simulink model "APB_Model0_v03_Test"  (R2020b)
settings: Solver=ode45  StartTime=0.0  StopTime=inf  RelTol=1e-3
undefined symbols (not defined in the file or in its folder): calb_Driver_acce, calb_Driver_bttn, calb_Driver_EmrBrk, calb_Driver_Prss, G_Fclamp, G_Kmot, G_Rmot, G_Stroke, G_SwOmega, GEN3, PbcDataStorageRequest_t
libraries: etargetslib x26, Lib_Op_Hndl x4, simulink x2, PbcOut_Checksum x2
(part 4 of 5)

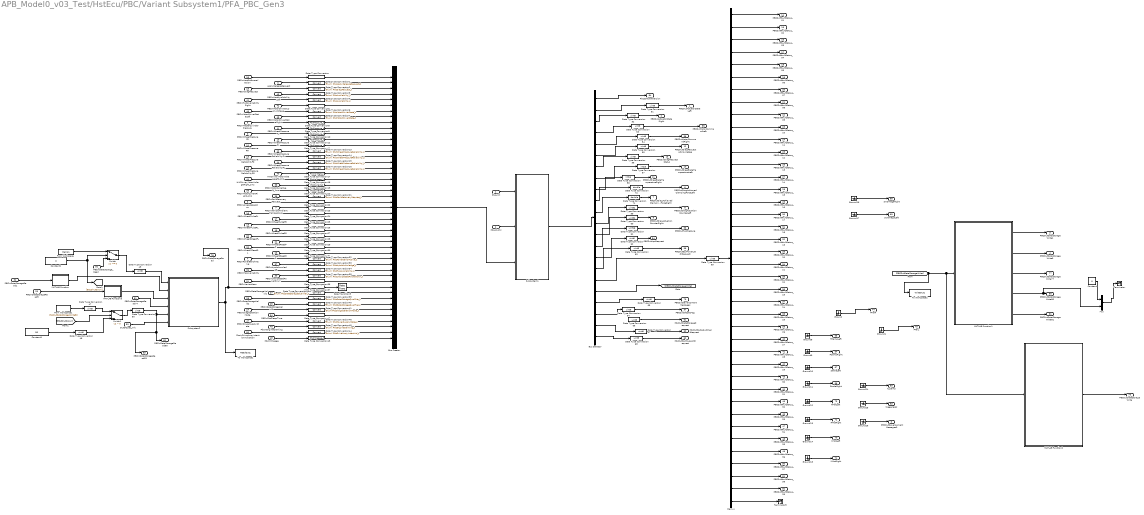
== system APB_Model0_v03_Test/HstEcu/PBC/Variant Subsystem1/PFA_PBC_Gen3 ==
  Pbc_Init : Inport
  Pbc_Cyclic : Inport  Port=2
  ApplyReleaseRequest : Inport  Port=3
      settings: AttributesFormatString=|
      | Type : %<OutDataTypeStr>
      | Unit : %<Unit>
  PBCInRollerBenchActive : Inport  Port=4
      settings: AttributesFormatString=|
      | Type : %<OutDataTypeStr>
      | Unit : %<Unit>
  PBCInLongAcceleration : Inport  Port=5
      settings: AttributesFormatString=|
      | Type : %<OutDataTypeStr>
      | Unit : %<Unit>
  PBCInMasterCylinderPressure : Inport  Port=6
      settings: AttributesFormatString=|
      | Type : %<OutDataTypeStr>
      | Unit : %<Unit>
  PBCInVehicleAmbientTemperature : Inport  Port=7
      settings: AttributesFormatString=|
      | Type : %<OutDataTypeStr>
      | Unit : %<Unit>
  PBCInWheelPressureFL : Inport  Port=8
      settings: AttributesFormatString=|
      | Type : %<OutDataTypeStr>
      | Unit : %<Unit>
  PBCInWheelPressureFR : Inport  Port=9
      settings: AttributesFormatString=|
      | Type : %<OutDataTypeStr>
      | Unit : %<Unit>
  PBCInWheelPressureRL : Inport  Port=10
      settings: AttributesFormatString=|
      | Type : %<OutDataTypeStr>
      | Unit : %<Unit>
  PBCInWheelPressureRR : Inport  Port=11
      settings: AttributesFormatString=|
      | Type : %<OutDataTypeStr>
      | Unit : %<Unit>
  PBCInWheelPressureReliabilityFL : Inport  Port=12
      settings: AttributesFormatString=|
      | Type : %<OutDataTypeStr>
      | Unit : %<Unit>
  PBCInWheelPressureReliabilityFR : Inport  Port=13
      settings: AttributesFormatString=|
      | Type : %<OutDataTypeStr>
      | Unit : %<Unit>
  PBCInWheelPressureReliabilityRL : Inport  Port=14
      settings: AttributesFormatString=|
      | Type : %<OutDataTypeStr>
      | Unit : %<Unit>
  PBCInWheelPressureReliabilityRR : Inport  Port=15
      settings: AttributesFormatString=|
      | Type : %<OutDataTypeStr>
      | Unit : %<Unit>
  PBCInWheelPulseFL : Inport  Port=16
      settings: AttributesFormatString=|
      | Type : %<OutDataTypeStr>
      | Unit : %<Unit>
  PBCInWheelPulseFR : Inport  Port=17
      settings: AttributesFormatString=|
      | Type : %<OutDataTypeStr>
      | Unit : %<Unit>
  PBCInWheelPulseRL : Inport  Port=18
      settings: AttributesFormatString=|
      | Type : %<OutDataTypeStr>
      | Unit : %<Unit>
  PBCInWheelPulseRR : Inport  Port=19
      settings: AttributesFormatString=|
      | Type : %<OutDataTypeStr>
      | Unit : %<Unit>
  PBCInWheelSPeedFL : Inport  Port=20
      settings: AttributesFormatString=|
      | Type : %<OutDataTypeStr>
      | Unit : %<Unit>
  PBCInWheelSPeedFR : Inport  Port=21
      settings: AttributesFormatString=|
      | Type : %<OutDataTypeStr>
      | Unit : %<Unit>
  PBCInWheelSPeedRL : Inport  Port=22
      settings: AttributesFormatString=|
      | Type : %<OutDataTypeStr>
      | Unit : %<Unit>
  PBCInWheelSPeedRR : Inport  Port=23
      settings: AttributesFormatString=|
      | Type : %<OutDataTypeStr>
      | Unit : %<Unit>
  PBCInDiagOperationMode : Inport  Port=24
      settings: AttributesFormatString=|
      | Type : %<OutDataTypeStr>
      | Unit : %<Unit>
  PBCInDiagRequest : Inport  Port=25
      settings: AttributesFormatString=|
      | Type : %<OutDataTypeStr>
      | Unit : %<Unit>
  PBCinHostSoftwareVersion : Inport  Port=26
      settings: AttributesFormatString=|
      | Type : %<OutDataTypeStr>
      | Unit : %<Unit>
  PBCInDataStorageValid1 : Inport  Port=27
      settings: AttributesFormatString=|
      | Type : %<OutDataTypeStr>
      | Unit : %<Unit>
  PBCInDataStorageValid2 : Inport  Port=28
      settings: AttributesFormatString=|
      | Type : %<OutDataTypeStr>
      | Unit : %<Unit>
  PBCInDataStorageValid3 : Inport  Port=29
      settings: AttributesFormatString=|
      | Type : %<OutDataTypeStr>
      | Unit : %<Unit>
  PBCInUnexpectedPowerDown : Inport  Port=30
      settings: AttributesFormatString=|
      | Type : %<OutDataTypeStr>
      | Unit : %<Unit>
  PBCInVariantItem : Inport  Port=31
      settings: AttributesFormatString=|
      | Type : %<OutDataTypeStr>
      | Unit : %<Unit>
  PBCInDataStorageRead1 : Inport  Port=32
      settings: AttributesFormatString=|
      | Type : %<OutDataTypeStr>
      | Unit : %<Unit>
  PBCInDataStorageRead9 : Inport  Port=33
      settings: AttributesFormatString=|
      | Type : %<OutDataTypeStr>
      | Unit : %<Unit>
  PBCInPbcSleepTime : Inport  Port=34
      settings: AttributesFormatString=|
      | Type : %<OutDataTypeStr>
      | Unit : %<Unit>
  PBCInFaultRecoveryRequest : Inport  Port=35
      settings: AttributesFormatString=|
      | Type : %<OutDataTypeStr>
      | Unit : %<Unit>
  PBCInHpsAvailability : Inport  Port=36
      settings: AttributesFormatString=|
      | Type : %<OutDataTypeStr>
      | Unit : %<Unit>
  PBCInHpsAcknowledge : Inport  Port=37
      settings: AttributesFormatString=|
      | Type : %<OutDataTypeStr>
      | Unit : %<Unit>
  PBCInMotorCurrentLeft_1ms : Inport  Port=38
      settings: AttributesFormatString=|
      | Type : %<OutDataTypeStr>
      | Unit : %<Unit>
  PBCInMotorCurrentRight_1ms : Inport  Port=39
      settings: AttributesFormatString=|
      | Type : %<OutDataTypeStr>
      | Unit : %<Unit>
  HWDriver_MotorVoltageLeft_1ms : Inport  Port=40
      settings: AttributesFormatString=|
      | Type : %<OutDataTypeStr>
      | Unit : %<Unit>
  HWDriver_MotorVoltageRight_1ms : Inport  Port=41
      settings: AttributesFormatString=|
      | Type : %<OutDataTypeStr>
      | Unit : %<Unit>
  PBCInMotorDriverSupplyVoltage : Inport  Port=42
      settings: AttributesFormatString=|
      | Type : %<OutDataTypeStr>
      | Unit : %<Unit>
  PBCinHostAvailabilityLeft : Inport  Port=43
      settings: AttributesFormatString=|
      | Type : %<OutDataTypeStr>
      | Unit : %<Unit>
  PBCinHostAvailabilityRight : Inport  Port=44
      settings: AttributesFormatString=|
      | Type : %<OutDataTypeStr>
      | Unit : %<Unit>
  PBCInMotorDriverStateLeft : Inport  Port=45
      settings: AttributesFormatString=|
      | Type : %<OutDataTypeStr>
      | Unit : %<Unit>
  PBCInMotorDriverStateRight : Inport  Port=46
      settings: AttributesFormatString=|
      | Type : %<OutDataTypeStr>
      | Unit : %<Unit>
  PBCInPowerSupplyState : Inport  Port=47
      settings: AttributesFormatString=|
      | Type : %<OutDataTypeStr>
      | Unit : %<Unit>
  PbcInMileage : Inport  Port=48
      settings: AttributesFormatString=|
      | Type : %<OutDataTypeStr>
      | Unit : %<Unit>
  PbcInEngineCranking : Inport  Port=49
      settings: AttributesFormatString=|
      | Type : %<OutDataTypeStr>
      | Unit : %<Unit>
  PbcInDriveAwayIntentionIndication : Inport  Port=50
      settings: AttributesFormatString=|
      | Type : %<OutDataTypeStr>
      | Unit : %<Unit>
  PBCInDataStorageRead77 : Inport  Port=51
      settings: AttributesFormatString=|
      | Type : %<OutDataTypeStr>
      | Unit : %<Unit>
  PBCInDataStorage_Read : Inport  Port=52
      settings: AttributesFormatString=|
      | Type : %<OutDataTypeStr>
      | Unit : %<Unit>
  OutOfSpec_Init : Inport  Port=53
  Bus Creator : BusCreator  Inputs=47  OutDataTypeStr=Bus: PbcIn_t  NonVirtualBus=on
  Bus Selector : BusSelector  OutputSignals=PbcSoftwareVersion,ActuatorStateLeft,ActuatorStateRight,MotorCommandLeft,MotorCommandRight,DiagRequestAcknowledge,DiagRequestStatus,DiagBrakeTemperatureLeft,DiagBrakeTemperatureRight,DiagAchievedClampForceLeft,DiagAchievedClampForceRight,DiagActuationCounterLeft,DiagActuationCounterRight,HpsPressure,HpsRequest,EcuPowerLatchRequest,FaultStatus,DataStorageWrite,DevelopmentMessages,OutOfSpecMsg,PadAdjustmentRequest,ParkSupportRequest
  Constant : Constant  Value=0
  Constant1 : Constant  Value=50
  Constant2 : Constant  Value=0
  Data Type Conversion : DataTypeConversion  OutDataTypeStr=PbcVersionChar_t
  Data Type Conversion1 : DataTypeConversion  OutDataTypeStr=Enum: PbcApplyReleaseRequest_t
  Data Type Conversion{8..12} (5 alike) : DataTypeConversion  OutDataTypeStr=PbcPressure_t
  Data Type Conversion{13..16} (4 alike) : DataTypeConversion  OutDataTypeStr=Enum: PbcWheelPressureReliability_t
  Data Type Conversion17 : DataTypeConversion  OutDataTypeStr=PbcVoltage_t
  Data Type Conversion18 : DataTypeConversion  OutDataTypeStr=PbcVoltage_t
  Data Type Conversion19 : DataTypeConversion  OutDataTypeStr=PbcCurrent_t
  Data Type Conversion2 : DataTypeConversion  OutDataTypeStr=Enum: PbcDiagRequest_t
  Data Type Conversion20 : DataTypeConversion  OutDataTypeStr=PbcCurrent_t
  Data Type Conversion21 : DataTypeConversion  OutDataTypeStr=Enum: PbcFaultRecoveryRequest_t
  Data Type Conversion22 : DataTypeConversion  OutDataTypeStr=PbcAcceleration_t
  Data Type Conversion23 : DataTypeConversion  OutDataTypeStr=PbcTemperature_t
  Data Type Conversion{24..27} (4 alike) : DataTypeConversion  OutDataTypeStr=PbcWheelPulse_t
  Data Type Conversion{28..31} (4 alike) : DataTypeConversion  OutDataTypeStr=PbcWheelSpeed_t
  Data Type Conversion3 : DataTypeConversion  OutDataTypeStr=Enum: PbcAvailability_t
  Data Type Conversion32 : DataTypeConversion  OutDataTypeStr=Enum: PbcRollerbenchActive_t
  Data Type Conversion33 : DataTypeConversion  OutDataTypeStr=Enum: PbcHpsAcknowledge_t
  Data Type Conversion34 : DataTypeConversion  OutDataTypeStr=Enum: PbcHpsAvailability_t
  Data Type Conversion35 : DataTypeConversion  OutDataTypeStr=Enum: PbcUnexpectedPowerdown_t
  Data Type Conversion36 : DataTypeConversion  OutDataTypeStr=PbcVariantItem_t
  Data Type Conversion37 : DataTypeConversion  OutDataTypeStr=PbcDataStorage_t
  Data Type Conversion38 : DataTypeConversion  OutDataTypeStr=Enum: PbcDataStorageQualifier_t
  Data Type Conversion39 : DataTypeConversion  OutDataTypeStr=Enum: PbcDataStorageQualifier_t
  Data Type Conversion4 : DataTypeConversion  OutDataTypeStr=Enum: PbcAvailability_t
  Data Type Conversion40 : DataTypeConversion  OutDataTypeStr=Enum: PbcDataStorageQualifier_t
  Data Type Conversion41 : DataTypeConversion  OutDataTypeStr=Enum:PbcDiagOperationMode_t
  Data Type Conversion42 : DataTypeConversion  OutDataTypeStr=PbcSleepTime_t
  Data Type Conversion43 : DataTypeConversion  OutDataTypeStr=PbcMileage_t
  Data Type Conversion44 : DataTypeConversion  OutDataTypeStr=Enum: PbcDriveAwayIntentInd_t
  Data Type Conversion45 : DataTypeConversion  OutDataTypeStr=Enum: PbcEngineCranking_t
  Data Type Conversion46 : DataTypeConversion  OutDataTypeStr=Enum: PbcPowerSupplyState_t
  Data Type Conversion{47..56,62..69} (18 alike) : DataTypeConversion  OutDataTypeStr=uint8
  Data Type Conversion5 : DataTypeConversion  OutDataTypeStr=PbcDriverVoltage_t
  Data Type Conversion57 : DataTypeConversion  OutDataTypeStr=int16
  Data Type Conversion58 : DataTypeConversion  OutDataTypeStr=int16
  Data Type Conversion59 : DataTypeConversion  OutDataTypeStr=uint32
  Data Type Conversion6 : DataTypeConversion  OutDataTypeStr=Enum: PbcMotorDriverState_t
  Data Type Conversion60 : DataTypeConversion  OutDataTypeStr=uint32
  Data Type Conversion61 : DataTypeConversion  OutDataTypeStr=uint16
  Data Type Conversion7 : DataTypeConversion  OutDataTypeStr=Enum: PbcMotorDriverState_t
  Data Type Conversion70 : DataTypeConversion  OutDataTypeStr=double
  Data Type Conversion71 : DataTypeConversion  OutDataTypeStr=double
  Demux : Demux  Outputs=40
  From Workspace : FromWorkspace  VariableName=Memo1
  From Workspace1 : FromWorkspace  VariableName=PbcOutDataStorageWrite80
  Ground{,1,8..17,24..26} (15 alike) : Ground
  MATLAB Function : MATLAB Function  TreatAsAtomicUnit=on
  MATLAB Function1 : MATLAB Function  TreatAsAtomicUnit=on
  MATLAB Function2 : MATLAB Function  TreatAsAtomicUnit=on
  MATLAB Function3 : MATLAB Function  TreatAsAtomicUnit=on
  Mux : Mux  Inputs=2
  Rate Transition5 : RateTransition  OutPortSampleTime=0.01
      settings: AttributesFormatString=%<OutPortSampleTime>
  Subsystem1 : Subsystem
  Subsystem2 : Subsystem
  Switch : Switch  Criteria=u2 ~= 0
  Switch1 : Switch  Criteria=u2 > Threshold
  Terminator : Terminator
  Terminator3 : Terminator
  To Workspace1 : ToWorkspace  VariableName=ReadOut1  SaveFormat=Timeseries  SampleTime=-1
  To Workspace2 : ToWorkspace  VariableName=WriteOut1  SaveFormat=Timeseries  SampleTime=-1
  PBCOutActuatorStateLeft : Outport  VectorParamsAs1DForOutWhenUnconnected=off
      settings: AttributesFormatString=|
      | Type : %<OutDataTypeStr>\nInit :%<InitialOutput>
      | Unit : %<Unit>
  PBCOutActuatorStateRight : Outport  Port=2  VectorParamsAs1DForOutWhenUnconnected=off
      settings: AttributesFormatString=|
      | Type : %<OutDataTypeStr>\nInit :%<InitialOutput>
      | Unit : %<Unit>
  PBCOutDataStorageWrite1 : Outport  Port=3  VectorParamsAs1DForOutWhenUnconnected=off
      settings: AttributesFormatString=|
      | Type : %<OutDataTypeStr>\nInit :%<InitialOutput>
      | Unit : %<Unit>
  PBCOutDataStorageWrite9 : Outport  Port=4  VectorParamsAs1DForOutWhenUnconnected=off
      settings: AttributesFormatString=|
      | Type : %<OutDataTypeStr>\nInit :%<InitialOutput>
      | Unit : %<Unit>
  PBCOutDevelopmentMessages0 : Outport  Port=5  VectorParamsAs1DForOutWhenUnconnected=off
      settings: AttributesFormatString=|
      | Type : %<OutDataTypeStr>\nInit :%<InitialOutput>
      | Unit : %<Unit>
  PBCOutDiagAchievedClampingForceLeft : Outport  Port=6  VectorParamsAs1DForOutWhenUnconnected=off
      settings: AttributesFormatString=|
      | Type : %<OutDataTypeStr>\nInit :%<InitialOutput>
      | Unit : %<Unit>
  PBCOutDiagAchievedClampingForceRight : Outport  Port=7  VectorParamsAs1DForOutWhenUnconnected=off
      settings: AttributesFormatString=|
      | Type : %<OutDataTypeStr>\nInit :%<InitialOutput>
      | Unit : %<Unit>
  PBCOutDiagActuationCounterLeft : Outport  Port=8  VectorParamsAs1DForOutWhenUnconnected=off
      settings: AttributesFormatString=|
      | Type : %<OutDataTypeStr>\nInit :%<InitialOutput>
      | Unit : %<Unit>
  PBCOutDiagActuationCounterRight : Outport  Port=9  VectorParamsAs1DForOutWhenUnconnected=off
      settings: AttributesFormatString=|
      | Type : %<OutDataTypeStr>\nInit :%<InitialOutput>
      | Unit : %<Unit>
  PBCOutDiagBrakeTemperatureLeft : Outport  Port=10  VectorParamsAs1DForOutWhenUnconnected=off
      settings: AttributesFormatString=|
      | Type : %<OutDataTypeStr>\nInit :%<InitialOutput>
      | Unit : %<Unit>
  PBCOutDiagBrakeTemperatureRight : Outport  Port=11  VectorParamsAs1DForOutWhenUnconnected=off
      settings: AttributesFormatString=|
      | Type : %<OutDataTypeStr>\nInit :%<InitialOutput>
      | Unit : %<Unit>
  PBCOutDiagRequestAcknowledge : Outport  Port=12  VectorParamsAs1DForOutWhenUnconnected=off
      settings: AttributesFormatString=|
      | Type : %<OutDataTypeStr>\nInit :%<InitialOutput>
      | Unit : %<Unit>
  PBCOutDiagRequestStatus : Outport  Port=13  VectorParamsAs1DForOutWhenUnconnected=off
      settings: AttributesFormatString=|
      | Type : %<OutDataTypeStr>\nInit :%<InitialOutput>
      | Unit : %<Unit>
  PBCOutFaultStatus_01 : Outport  Port=14  VectorParamsAs1DForOutWhenUnconnected=off
      settings: AttributesFormatString=|
      | Type : %<OutDataTypeStr>\nInit :%<InitialOutput>
      | Unit : %<Unit>
  PBCOutFaultStatus_02 : Outport  Port=15  VectorParamsAs1DForOutWhenUnconnected=off
      settings: AttributesFormatString=|
      | Type : %<OutDataTypeStr>\nInit :%<InitialOutput>
      | Unit : %<Unit>
  PBCOutFaultStatus_03 : Outport  Port=16  VectorParamsAs1DForOutWhenUnconnected=off
      settings: AttributesFormatString=|
      | Type : %<OutDataTypeStr>\nInit :%<InitialOutput>
      | Unit : %<Unit>
  PBCOutFaultStatus_04 : Outport  Port=17  VectorParamsAs1DForOutWhenUnconnected=off
      settings: AttributesFormatString=|
      | Type : %<OutDataTypeStr>\nInit :%<InitialOutput>
      | Unit : %<Unit>
  PBCOutFaultStatus_05 : Outport  Port=18  VectorParamsAs1DForOutWhenUnconnected=off
      settings: AttributesFormatString=|
      | Type : %<OutDataTypeStr>\nInit :%<InitialOutput>
      | Unit : %<Unit>
  PBCOutFaultStatus_06 : Outport  Port=19  VectorParamsAs1DForOutWhenUnconnected=off
      settings: AttributesFormatString=|
      | Type : %<OutDataTypeStr>\nInit :%<InitialOutput>
      | Unit : %<Unit>
  PBCOutFaultStatus_07 : Outport  Port=20  VectorParamsAs1DForOutWhenUnconnected=off
      settings: AttributesFormatString=|
      | Type : %<OutDataTypeStr>\nInit :%<InitialOutput>
      | Unit : %<Unit>
  PBCOutFaultStatus_08 : Outport  Port=21  VectorParamsAs1DForOutWhenUnconnected=off
      settings: AttributesFormatString=|
      | Type : %<OutDataTypeStr>\nInit :%<InitialOutput>
      | Unit : %<Unit>
  PBCOutFaultStatus_09 : Outport  Port=22  VectorParamsAs1DForOutWhenUnconnected=off
      settings: AttributesFormatString=|
      | Type : %<OutDataTypeStr>\nInit :%<InitialOutput>
      | Unit : %<Unit>
  PBCOutFaultStatus_10 : Outport  Port=23  VectorParamsAs1DForOutWhenUnconnected=off
      settings: AttributesFormatString=|
      | Type : %<OutDataTypeStr>\nInit :%<InitialOutput>
      | Unit : %<Unit>
  PBCOutFaultStatus_11 : Outport  Port=24  VectorParamsAs1DForOutWhenUnconnected=off
      settings: AttributesFormatString=|
      | Type : %<OutDataTypeStr>\nInit :%<InitialOutput>
      | Unit : %<Unit>
  PBCOutFaultStatus_12 : Outport  Port=25  VectorParamsAs1DForOutWhenUnconnected=off
      settings: AttributesFormatString=|
      | Type : %<OutDataTypeStr>\nInit :%<InitialOutput>
      | Unit : %<Unit>
  PBCOutFaultStatus_13 : Outport  Port=26  VectorParamsAs1DForOutWhenUnconnected=off
      settings: AttributesFormatString=|
      | Type : %<OutDataTypeStr>\nInit :%<InitialOutput>
      | Unit : %<Unit>
  PBCOutFaultStatus_14 : Outport  Port=27  VectorParamsAs1DForOutWhenUnconnected=off
      settings: AttributesFormatString=|
      | Type : %<OutDataTypeStr>\nInit :%<InitialOutput>
      | Unit : %<Unit>
  PBCOutFaultStatus_15 : Outport  Port=28  VectorParamsAs1DForOutWhenUnconnected=off
      settings: AttributesFormatString=|
      | Type : %<OutDataTypeStr>\nInit :%<InitialOutput>
      | Unit : %<Unit>
  PBCOutFaultStatus_16 : Outport  Port=29  VectorParamsAs1DForOutWhenUnconnected=off
      settings: AttributesFormatString=|
      | Type : %<OutDataTypeStr>\nInit :%<InitialOutput>
      | Unit : %<Unit>
  PBCOutFaultStatus_17 : Outport  Port=30  VectorParamsAs1DForOutWhenUnconnected=off
      settings: AttributesFormatString=|
      | Type : %<OutDataTypeStr>\nInit :%<InitialOutput>
      | Unit : %<Unit>
  PBCOutFaultStatus_18 : Outport  Port=31  VectorParamsAs1DForOutWhenUnconnected=off
      settings: AttributesFormatString=|
      | Type : %<OutDataTypeStr>\nInit :%<InitialOutput>
      | Unit : %<Unit>
  PBCOutFaultStatus_19 : Outport  Port=32  VectorParamsAs1DForOutWhenUnconnected=off
      settings: AttributesFormatString=|
      | Type : %<OutDataTypeStr>\nInit :%<InitialOutput>
      | Unit : %<Unit>
  PBCOutFaultStatus_20 : Outport  Port=33  VectorParamsAs1DForOutWhenUnconnected=off
      settings: AttributesFormatString=|
      | Type : %<OutDataTypeStr>\nInit :%<InitialOutput>
      | Unit : %<Unit>
  PBCOutFaultStatus_21 : Outport  Port=34  VectorParamsAs1DForOutWhenUnconnected=off
      settings: AttributesFormatString=|
      | Type : %<OutDataTypeStr>\nInit :%<InitialOutput>
      | Unit : %<Unit>
  PBCOutFaultStatus_22 : Outport  Port=35  VectorParamsAs1DForOutWhenUnconnected=off
      settings: AttributesFormatString=|
      | Type : %<OutDataTypeStr>\nInit :%<InitialOutput>
      | Unit : %<Unit>
  PBCOutFaultStatus_23 : Outport  Port=36  VectorParamsAs1DForOutWhenUnconnected=off
      settings: AttributesFormatString=|
      | Type : %<OutDataTypeStr>\nInit :%<InitialOutput>
      | Unit : %<Unit>
  PBCOutFaultStatus_24 : Outport  Port=37  VectorParamsAs1DForOutWhenUnconnected=off
      settings: AttributesFormatString=|
      | Type : %<OutDataTypeStr>\nInit :%<InitialOutput>
      | Unit : %<Unit>
  PBCOutFaultStatus_25 : Outport  Port=38  VectorParamsAs1DForOutWhenUnconnected=off
      settings: AttributesFormatString=|
      | Type : %<OutDataTypeStr>\nInit :%<InitialOutput>
      | Unit : %<Unit>
  PBCOutFaultStatus_26 : Outport  Port=39  VectorParamsAs1DForOutWhenUnconnected=off
      settings: AttributesFormatString=|
      | Type : %<OutDataTypeStr>\nInit :%<InitialOutput>
      | Unit : %<Unit>
  PBCOutFaultStatus_27 : Outport  Port=40  VectorParamsAs1DForOutWhenUnconnected=off
      settings: AttributesFormatString=|
      | Type : %<OutDataTypeStr>\nInit :%<InitialOutput>
      | Unit : %<Unit>
  PBCOutFaultStatus_28 : Outport  Port=41  VectorParamsAs1DForOutWhenUnconnected=off
      settings: AttributesFormatString=|
      | Type : %<OutDataTypeStr>\nInit :%<InitialOutput>
      | Unit : %<Unit>
  PBCOutFaultStatus_29 : Outport  Port=42  VectorParamsAs1DForOutWhenUnconnected=off
      settings: AttributesFormatString=|
      | Type : %<OutDataTypeStr>\nInit :%<InitialOutput>
      | Unit : %<Unit>
  PBCOutFaultStatus_30 : Outport  Port=43  VectorParamsAs1DForOutWhenUnconnected=off
      settings: AttributesFormatString=|
      | Type : %<OutDataTypeStr>\nInit :%<InitialOutput>
      | Unit : %<Unit>
  PBCOutFaultStatus_31 : Outport  Port=44  VectorParamsAs1DForOutWhenUnconnected=off
      settings: AttributesFormatString=|
      | Type : %<OutDataTypeStr>\nInit :%<InitialOutput>
      | Unit : %<Unit>
  PBCOutFaultStatus_32 : Outport  Port=45  VectorParamsAs1DForOutWhenUnconnected=off
      settings: AttributesFormatString=|
      | Type : %<OutDataTypeStr>\nInit :%<InitialOutput>
      | Unit : %<Unit>
  PBCOutFaultStatus_33 : Outport  Port=46  VectorParamsAs1DForOutWhenUnconnected=off
      settings: AttributesFormatString=|
      | Type : %<OutDataTypeStr>\nInit :%<InitialOutput>
      | Unit : %<Unit>
  PBCOutFaultStatus_34 : Outport  Port=47  VectorParamsAs1DForOutWhenUnconnected=off
      settings: AttributesFormatString=|
      | Type : %<OutDataTypeStr>\nInit :%<InitialOutput>
      | Unit : %<Unit>
  PBCOutFaultStatus_35 : Outport  Port=48  VectorParamsAs1DForOutWhenUnconnected=off
      settings: AttributesFormatString=|
      | Type : %<OutDataTypeStr>\nInit :%<InitialOutput>
      | Unit : %<Unit>
  PBCOutFaultStatus_36 : Outport  Port=49  VectorParamsAs1DForOutWhenUnconnected=off
      settings: AttributesFormatString=|
      | Type : %<OutDataTypeStr>\nInit :%<InitialOutput>
      | Unit : %<Unit>
  PBCOutFaultStatus_37 : Outport  Port=50  VectorParamsAs1DForOutWhenUnconnected=off
      settings: AttributesFormatString=|
      | Type : %<OutDataTypeStr>\nInit :%<InitialOutput>
      | Unit : %<Unit>
  PBCOutFaultStatus_38 : Outport  Port=51  VectorParamsAs1DForOutWhenUnconnected=off
      settings: AttributesFormatString=|
      | Type : %<OutDataTypeStr>\nInit :%<InitialOutput>
      | Unit : %<Unit>
  PBCOutFaultStatus_39 : Outport  Port=52  VectorParamsAs1DForOutWhenUnconnected=off
      settings: AttributesFormatString=|
      | Type : %<OutDataTypeStr>\nInit :%<InitialOutput>
      | Unit : %<Unit>
  PBCOutHpsPressure : Outport  Port=53  VectorParamsAs1DForOutWhenUnconnected=off
      settings: AttributesFormatString=|
      | Type : %<OutDataTypeStr>\nInit :%<InitialOutput>
      | Unit : %<Unit>
  PBCOutHpsRequest : Outport  Port=54  VectorParamsAs1DForOutWhenUnconnected=off
      settings: AttributesFormatString=|
      | Type : %<OutDataTypeStr>\nInit :%<InitialOutput>
      | Unit : %<Unit>
  PBCOutMotorCommandLeft : Outport  Port=55  VectorParamsAs1DForOutWhenUnconnected=off
      settings: AttributesFormatString=|
      | Type : %<OutDataTypeStr>\nInit :%<InitialOutput>
      | Unit : %<Unit>
  PBCOutMotorCommandRight : Outport  Port=56  VectorParamsAs1DForOutWhenUnconnected=off
      settings: AttributesFormatString=|
      | Type : %<OutDataTypeStr>\nInit :%<InitialOutput>
      | Unit : %<Unit>
  PBCOutOfSpecMsg : Outport  Port=57  VectorParamsAs1DForOutWhenUnconnected=off
      settings: AttributesFormatString=|
      | Type : %<OutDataTypeStr>\nInit :%<InitialOutput>
      | Unit : %<Unit>
  PBCOutEcuPowerLatchRequest : Outport  Port=58  VectorParamsAs1DForOutWhenUnconnected=off
      settings: AttributesFormatString=|
      | Type : %<OutDataTypeStr>\nInit :%<InitialOutput>
      | Unit : %<Unit>
  F_clamp : Outport  Port=59  VectorParamsAs1DForOutWhenUnconnected=off
      settings: AttributesFormatString=|
      | Type : %<OutDataTypeStr>\nInit :%<InitialOutput>
      | Unit : %<Unit>
  PbcOutPadAdjustmentRequest : Outport  Port=60  VectorParamsAs1DForOutWhenUnconnected=off
      settings: AttributesFormatString=|
      | Type : %<OutDataTypeStr>\nInit :%<InitialOutput>
      | Unit : %<Unit>
  PbcOutDataStorageRequest : Outport  Port=61  VectorParamsAs1DForOutWhenUnconnected=off
      settings: AttributesFormatString=|
      | Type : %<OutDataTypeStr>\nInit :%<InitialOutput>
      | Unit : %<Unit>
  PbcOutParkSupportRequest : Outport  Port=62  VectorParamsAs1DForOutWhenUnconnected=off
      settings: AttributesFormatString=|
      | Type : %<OutDataTypeStr>\nInit :%<InitialOutput>
      | Unit : %<Unit>
  triggerrecal : Outport  Port=63  VectorParamsAs1DForOutWhenUnconnected=off
      settings: AttributesFormatString=|
      | Type : %<OutDataTypeStr>\nInit :%<InitialOutput>
      | Unit : %<Unit>
  FclampRight : Outport  Port=64  VectorParamsAs1DForOutWhenUnconnected=off
      settings: AttributesFormatString=|
      | Type : %<OutDataTypeStr>\nInit :%<InitialOutput>
      | Unit : %<Unit>
  FclampLeft : Outport  Port=65  VectorParamsAs1DForOutWhenUnconnected=off
      settings: AttributesFormatString=|
      | Type : %<OutDataTypeStr>\nInit :%<InitialOutput>
      | Unit : %<Unit>
  StrokeRight : Outport  Port=66  VectorParamsAs1DForOutWhenUnconnected=off
      settings: AttributesFormatString=|
      | Type : %<OutDataTypeStr>\nInit :%<InitialOutput>
      | Unit : %<Unit>
  StrokeLeft : Outport  Port=67  VectorParamsAs1DForOutWhenUnconnected=off
      settings: AttributesFormatString=|
      | Type : %<OutDataTypeStr>\nInit :%<InitialOutput>
      | Unit : %<Unit>
  SwOmegaRight : Outport  Port=68  VectorParamsAs1DForOutWhenUnconnected=off
      settings: AttributesFormatString=|
      | Type : %<OutDataTypeStr>\nInit :%<InitialOutput>
      | Unit : %<Unit>
  SwOmegaLeft : Outport  Port=69  VectorParamsAs1DForOutWhenUnconnected=off
      settings: AttributesFormatString=|
      | Type : %<OutDataTypeStr>\nInit :%<InitialOutput>
      | Unit : %<Unit>
  KMotLeft : Outport  Port=70  VectorParamsAs1DForOutWhenUnconnected=off
      settings: AttributesFormatString=|
      | Type : %<OutDataTypeStr>\nInit :%<InitialOutput>
      | Unit : %<Unit>
  KMotRight : Outport  Port=71  VectorParamsAs1DForOutWhenUnconnected=off
      settings: AttributesFormatString=|
      | Type : %<OutDataTypeStr>\nInit :%<InitialOutput>
      | Unit : %<Unit>
  RMotRight : Outport  Port=72  VectorParamsAs1DForOutWhenUnconnected=off
      settings: AttributesFormatString=|
      | Type : %<OutDataTypeStr>\nInit :%<InitialOutput>
      | Unit : %<Unit>
  RMotLeft : Outport  Port=73  VectorParamsAs1DForOutWhenUnconnected=off
      settings: AttributesFormatString=|
      | Type : %<OutDataTypeStr>\nInit :%<InitialOutput>
      | Unit : %<Unit>
  FTarR : Outport  Port=74
  FTarL : Outport  Port=75
  PBCOutDataStorageWrite : Outport  Port=76  VectorParamsAs1DForOutWhenUnconnected=off
      settings: AttributesFormatString=|
      | Type : %<OutDataTypeStr>\nInit :%<InitialOutput>
      | Unit : %<Unit>
  PBCOutDataStorageWrite77 : Outport  Port=77  VectorParamsAs1DForOutWhenUnconnected=off
      settings: AttributesFormatString=|
      | Type : %<OutDataTypeStr>\nInit :%<InitialOutput>
      | Unit : %<Unit>
  PBCInDataStorageRead : Outport  Port=78
  PBCOutDevelopmentMessages : Outport  Port=79  VectorParamsAs1DForOutWhenUnconnected=off
      settings: AttributesFormatString=|
      | Type : %<OutDataTypeStr>\nInit :%<InitialOutput>
      | Unit : %<Unit>
  PBCOutDataStorageWrite80 : Outport  Port=80  VectorParamsAs1DForOutWhenUnconnected=off
      settings: AttributesFormatString=|
      | Type : %<OutDataTypeStr>\nInit :%<InitialOutput>
      | Unit : %<Unit>
  PBCOutDataStorageWrite81 : Outport  Port=81  VectorParamsAs1DForOutWhenUnconnected=off
      settings: AttributesFormatString=|
      | Type : %<OutDataTypeStr>\nInit :%<InitialOutput>
      | Unit : %<Unit>
  PBCInDataStorageRead80 : Outport  Port=82  VectorParamsAs1DForOutWhenUnconnected=off
      settings: AttributesFormatString=|
      | Type : %<OutDataTypeStr>\nInit :%<InitialOutput>
      | Unit : %<Unit>
  PBCInDataStorageRead81 : Outport  Port=83  VectorParamsAs1DForOutWhenUnconnected=off
      settings: AttributesFormatString=|
      | Type : %<OutDataTypeStr>\nInit :%<InitialOutput>
      | Unit : %<Unit>
  PbcSoftwareVersion : Outport  Port=84
  wires:
  PBCInWheelPressureRR/1 -> Data Type Conversion11/1
  PBCInWheelPressureFL/1 -> Data Type Conversion9/1
  Data Type Conversion11/1 -> Bus Creator/13  "WheelPressureRearRight"
  Demux/35 -> PBCOutFaultStatus_35/1
  Demux/4 -> PBCOutFaultStatus_04/1
  Data Type Conversion8/1 -> Bus Creator/9  "MasterCylinderPressure"
  Data Type Conversion3/1 -> Bus Creator/4  "HostAvailabilityLeft"
  Data Type Conversion25/1 -> Bus Creator/26  "WheelPulseFrontRight"
  Bus Selector/5 -> Data Type Conversion54/1  "<MotorCommandRight>"
  MATLAB Function1/5(PBCOutDataStorageWrite81) -> PBCOutDataStorageWrite81/1
  Demux/40 -> Terminator3/1
  Demux/30 -> PBCOutFaultStatus_30/1
  PBCInPowerSupplyState/1 -> Data Type Conversion46/1
  MATLAB Function1/4(PBCOutDataStorageWrite80) -> Mux/2, PBCOutDataStorageWrite80/1
  Data Type Conversion21/1 -> Bus Creator/22  "FaultRecoveryRequest"
  PBCInWheelPressureReliabilityRL/1 -> Data Type Conversion15/1
  Bus Selector/13 -> Data Type Conversion60/1  "<DiagActuationCounterRight>"
  [PBCOutDataStorageWrite] -> To Workspace2/1, MATLAB Function1/1(PBCOutDataStorageWrite), MATLAB Function2/1(PBCOutDataStorageWrite)
  PBCInPbcSleepTime/1 -> Data Type Conversion42/1
  Ground24/1 -> F_clamp/1
  Ground26/1 -> PBCOutDevelopmentMessages0/1
  MATLAB Function1/1(PBCOutDataStorageWrite1) -> PBCOutDataStorageWrite1/1
  PBCInUnexpectedPowerDown/1 -> Data Type Conversion35/1
  Data Type Conversion19/1 -> Bus Creator/20  "MotorCurrentLeft"
  Demux/34 -> PBCOutFaultStatus_34/1
  Data Type Conversion28/1 -> Bus Creator/29  "WheelSpeedFrontLeft"
  Demux/10 -> PBCOutFaultStatus_10/1
  Data Type Conversion2/1 -> Bus Creator/3  "DiagRequest"
  PBCInVehicleAmbientTemperature/1 -> Data Type Conversion23/1
  Data Type Conversion31/1 -> Bus Creator/32  "WheelSpeedRearRight"
  HWDriver_MotorVoltageLeft_1ms/1 -> Data Type Conversion17/1
  Demux/31 -> PBCOutFaultStatus_31/1
  Demux/14 -> PBCOutFaultStatus_14/1
  PBCinHostSoftwareVersion/1 -> Data Type Conversion/1
  Demux/1 -> PBCOutFaultStatus_01/1
  Ground16/1 -> SwOmegaRight/1
  Ground14/1 -> KMotLeft/1
  Data Type Conversion41/1 -> Bus Creator/42  "DiagOperationMode"
  MATLAB Function1/3(PBCOutDataStorageWrite77) -> PBCOutDataStorageWrite77/1
  Demux/2 -> PBCOutFaultStatus_02/1
  Demux/29 -> PBCOutFaultStatus_29/1
  Bus Selector/3 -> Data Type Conversion52/1  "<ActuatorStateRight>"
  Ground17/1 -> SwOmegaLeft/1
  PBCInWheelPressureReliabilityRR/1 -> Data Type Conversion16/1
  Data Type Conversion38/1 -> Bus Creator/39  "DataStorageValid1"
  Ground15/1 -> KMotRight/1
  Ground8/1 -> FclampLeft/1
  Demux/36 -> PBCOutFaultStatus_36/1
  HWDriver_MotorVoltageRight_1ms/1 -> Data Type Conversion18/1
  Bus Selector/20 -> Data Type Conversion64/1  "<OutOfSpecMsg>"
  Data Type Conversion/1 -> Bus Creator/1  "HostSoftwareVersion"
  Demux/21 -> PBCOutFaultStatus_21/1
  Ground9/1 -> FclampRight/1
  Ground10/1 -> StrokeLeft/1
  Data Type Conversion50/1 -> Subsystem2/5(TDiscInit), PBCInDataStorageRead81/1, PBCInDataStorageRead80/1
  Demux/3 -> PBCOutFaultStatus_03/1
  Data Type Conversion65/1 -> PBCOutDevelopmentMessages/1
  Ground13/1 -> RMotRight/1
  From Workspace1/1 -> Data Type Conversion47/1
  Data Type Conversion30/1 -> Bus Creator/31  "WheelSpeedRearLeft"
  Data Type Conversion59/1 -> PBCOutDiagActuationCounterLeft/1
  Data Type Conversion35/1 -> Bus Creator/36  "UnexpectedPowerdown"
  Demux/8 -> PBCOutFaultStatus_08/1
  Bus Selector/10 -> Data Type Conversion70/1  "<DiagAchievedClampForceLeft>"
  Data Type Conversion58/1 -> PBCOutDiagBrakeTemperatureRight/1
  Subsystem1/1(PbcOut) -> Bus Selector/1
  Data Type Conversion47/1 -> Switch1/1
  Demux/27 -> PBCOutFaultStatus_27/1
  Data Type Conversion61/1 -> PBCOutHpsPressure/1
  Data Type Conversion20/1 -> Bus Creator/21  "MotorCurrentRight"
  Bus Selector/22 -> Data Type Conversion68/1  "<ParkSupportRequest>"
  Data Type Conversion6/1 -> Bus Creator/7  "MotorDriverStateLeft"
  Bus Selector/16 -> Data Type Conversion63/1  "<EcuPowerLatchRequest>"
  Data Type Conversion55/1 -> PBCOutDiagRequestAcknowledge/1
  Data Type Conversion54/1 -> PBCOutMotorCommandRight/1
  Bus Selector/2 -> Data Type Conversion51/1  "<ActuatorStateLeft>"
  Bus Selector/19 -> Data Type Conversion65/1  "<DevelopmentMessages>"
  PbcInDriveAwayIntentionIndication/1 -> Data Type Conversion44/1
  [ECUShutDown] -> Switch1/2
  Data Type Conversion49/1 -> Subsystem2/1(PBCInDataStorageRead)
  Demux/17 -> PBCOutFaultStatus_17/1
  PBCInMotorCurrentLeft_1ms/1 -> Data Type Conversion19/1
  MATLAB Function3/1(y) -> Subsystem2/3(PBCInDataStorageRead9_ActrSttRgt)
  Data Type Conversion51/1 -> PBCOutActuatorStateLeft/1
  Bus Selector/6 -> Data Type Conversion55/1  "<DiagRequestAcknowledge>"
  Data Type Conversion52/1 -> PBCOutActuatorStateRight/1
  PBCInLongAcceleration/1 -> Data Type Conversion22/1
  Demux/25 -> PBCOutFaultStatus_25/1
  Rate Transition5/1 -> Bus Creator/38  "DataStorageRead"
  Ground12/1 -> RMotLeft/1
  Mux/1 -> Terminator/1
  Ground1/1 -> FTarL/1
  Bus Selector/15 -> Data Type Conversion62/1  "<HpsRequest>"
  Demux/38 -> PBCOutFaultStatus_38/1
  Constant/1 -> Mux/1
  Data Type Conversion4/1 -> Bus Creator/5  "HostAvailabilityRight"
  Demux/39 -> PBCOutFaultStatus_39/1
  Switch1/1 -> Data Type Conversion50/1
  Bus Selector/1 -> PbcSoftwareVersion/1  "<PbcSoftwareVersion>"
  PBCInDataStorageValid2/1 -> Data Type Conversion39/1
  Bus Selector/7 -> Data Type Conversion56/1  "<DiagRequestStatus>"
  Data Type Conversion48/1 -> Switch1/3
  Switch/1 -> Data Type Conversion49/1
  Demux/13 -> PBCOutFaultStatus_13/1
  Data Type Conversion7/1 -> Bus Creator/8  "MotorDriverStateRight"
  PBCInDataStorage_Read/1 -> Switch/3
  MATLAB Function2/1(PBCOutDataStorageWrite_MIL) -> PBCOutDataStorageWrite/1
  Constant1/1 -> Data Type Conversion48/1
  Demux/20 -> PBCOutFaultStatus_20/1
  Pbc_Init/1 -> Subsystem1/1(Pbc_Init)
  PBCInWheelPressureReliabilityFR/1 -> Data Type Conversion14/1
  PBCInWheelPressureRL/1 -> Data Type Conversion12/1
  Data Type Conversion17/1 -> Bus Creator/18  "MotorVoltageLeft"
  From Workspace/1 -> Switch/1
  Demux/37 -> PBCOutFaultStatus_37/1
  Data Type Conversion46/1 -> Bus Creator/44  "PowerSupplyState"
  PBCinHostAvailabilityRight/1 -> Data Type Conversion4/1
  PBCInDiagOperationMode/1 -> Data Type Conversion41/1
  Bus Selector/17 -> Data Type Conversion69/1  "<FaultStatus>"
  PBCInWheelSPeedRL/1 -> Data Type Conversion30/1
  Pbc_Cyclic/1 -> Subsystem1/2(Pbc_Cyclic)
  PBCInDiagRequest/1 -> Data Type Conversion2/1
  Data Type Conversion15/1 -> Bus Creator/16  "WheelPressureReliabilityRearLeft"
  Demux/19 -> PBCOutFaultStatus_19/1
  Bus Selector/8 -> Data Type Conversion57/1  "<DiagBrakeTemperatureLeft>"
  Demux/33 -> PBCOutFaultStatus_33/1
  Demux/22 -> PBCOutFaultStatus_22/1
  Data Type Conversion16/1 -> Bus Creator/17  "WheelPressureReliabilityRearRight"
  PBCInDataStorageRead9/1 -> MATLAB Function3/1(u)
  Demux/5 -> PBCOutFaultStatus_05/1
  Demux/6 -> PBCOutFaultStatus_06/1
  Demux/26 -> PBCOutFaultStatus_26/1
  Bus Selector/11 -> Data Type Conversion71/1  "<DiagAchievedClampForceRight>"
  Data Type Conversion34/1 -> Bus Creator/35  "HpsAvailability"
  Demux/18 -> PBCOutFaultStatus_18/1
  Data Type Conversion44/1 -> Bus Creator/46  "DriveAwayIntentionIndication"
  Ground11/1 -> StrokeRight/1
  Bus Selector/9 -> Data Type Conversion58/1  "<DiagBrakeTemperatureRight>"
  PBCInWheelPulseFR/1 -> Data Type Conversion25/1
  PBCInWheelPressureReliabilityFL/1 -> Data Type Conversion13/1
  Data Type Conversion45/1 -> Bus Creator/45  "EngineCranking"
  Bus Selector/4 -> Data Type Conversion53/1  "<MotorCommandLeft>"
  Bus Selector/18 -> [PBCOutDataStorageWrite]  "<DataStorageWrite>"
  PBCInFaultRecoveryRequest/1 -> Data Type Conversion21/1
  Data Type Conversion27/1 -> Bus Creator/28  "WheelPulseRearRight"
  PBCInDataStorageValid3/1 -> Data Type Conversion40/1
  ApplyReleaseRequest/1 -> Data Type Conversion1/1
  PBCInHpsAvailability/1 -> Data Type Conversion34/1
  Data Type Conversion43/1 -> Bus Creator/47  "Mileage"
  Data Type Conversion39/1 -> Bus Creator/40  "DataStorageValid2"
  Demux/23 -> PBCOutFaultStatus_23/1
  PBCInDataStorageRead77/1 -> Subsystem2/4(PBCInDataStorageRead77)
  PBCInMasterCylinderPressure/1 -> Data Type Conversion8/1
  PbcInMileage/1 -> Data Type Conversion43/1
  Data Type Conversion40/1 -> Bus Creator/41  "DataStorageValid3"
  Data Type Conversion22/1 -> Bus Creator/23  "LongAcceleration"
  PBCInWheelPressureFR/1 -> Data Type Conversion10/1
  Data Type Conversion18/1 -> Bus Creator/19  "MotorVoltageRight"
  Data Type Conversion5/1 -> Bus Creator/6  "MotorDriverSupplyVoltage"
  Data Type Conversion29/1 -> Bus Creator/30  "WheelSpeedFrontRight"
  Data Type Conversion23/1 -> Bus Creator/24  "VehicleAmbientTemperature"
  Subsystem2/1(DataStorageRead) -> To Workspace1/1, PBCInDataStorageRead/1, Data Type Conversion37/1
  PBCInWheelPulseRL/1 -> Data Type Conversion26/1
  PBCInWheelSPeedRR/1 -> Data Type Conversion31/1
  PBCInWheelPulseRR/1 -> Data Type Conversion27/1
  Data Type Conversion42/1 -> Bus Creator/43  "PbcSleepTime"
  PBCInWheelSPeedFL/1 -> Data Type Conversion28/1
  Data Type Conversion56/1 -> PBCOutDiagRequestStatus/1
  PBCInVariantItem/1 -> Data Type Conversion36/1
  Data Type Conversion10/1 -> Bus Creator/11  "WheelPressureFrontRight"
  PBCInMotorCurrentRight_1ms/1 -> Data Type Conversion20/1
  MATLAB Function1/2(PBCOutDataStorageWrite9) -> PBCOutDataStorageWrite9/1
  Demux/15 -> PBCOutFaultStatus_15/1
  Data Type Conversion33/1 -> Bus Creator/34  "HpsAcknowledge"
  OutOfSpec_Init/1 -> Subsystem2/6(OutOfSpec_Init)
  Data Type Conversion37/1 -> Rate Transition5/1  "DataStorageRead"
  Data Type Conversion1/1 -> Bus Creator/2  "ApplyReleaseRequest"
  PBCInWheelPulseFL/1 -> Data Type Conversion24/1
  Data Type Conversion66/1 -> PbcOutDataStorageRequest/1
  Demux/7 -> PBCOutFaultStatus_07/1
  Demux/24 -> PBCOutFaultStatus_24/1
  Data Type Conversion63/1 -> PBCOutEcuPowerLatchRequest/1
  Demux/9 -> PBCOutFaultStatus_09/1
  MATLAB Function/1(y) -> Subsystem2/2(PBCInDataStorageRead1_ActrSttLft)
  Data Type Conversion12/1 -> Bus Creator/12  "WheelPressureRearLeft"
  PBCInWheelSPeedFR/1 -> Data Type Conversion29/1
  Data Type Conversion69/1 -> Demux/1
  Demux/11 -> PBCOutFaultStatus_11/1
  Data Type Conversion67/1 -> PbcOutPadAdjustmentRequest/1
  Data Type Conversion62/1 -> PBCOutHpsRequest/1
  PBCInDataStorageValid1/1 -> Data Type Conversion38/1
  Data Type Conversion60/1 -> PBCOutDiagActuationCounterRight/1
  Demux/16 -> PBCOutFaultStatus_16/1
  PbcInEngineCranking/1 -> Data Type Conversion45/1
  Data Type Conversion70/1 -> PBCOutDiagAchievedClampingForceLeft/1
  Data Type Conversion71/1 -> PBCOutDiagAchievedClampingForceRight/1
  Data Type Conversion9/1 -> Bus Creator/10  "WheelPressureFrontLeft"
  Data Type Conversion57/1 -> PBCOutDiagBrakeTemperatureLeft/1
  Bus Selector/21 -> Data Type Conversion67/1  "<PadAdjustmentRequest>"
  Bus Selector/14 -> Data Type Conversion61/1  "<HpsPressure>"
  Data Type Conversion68/1 -> PbcOutParkSupportRequest/1
  Data Type Conversion32/1 -> Bus Creator/33  "RollerbenchActive"
  PBCinHostAvailabilityLeft/1 -> Data Type Conversion3/1
  Constant2/1 -> [ECUShutDown], Switch/2
  PBCInMotorDriverSupplyVoltage/1 -> Data Type Conversion5/1
  Ground25/1 -> triggerrecal/1
  PBCInMotorDriverStateRight/1 -> Data Type Conversion7/1
  ? -> Data Type Conversion66/1  "<StorageRequest>"
  Data Type Conversion36/1 -> Bus Creator/37  "VariantItem"
  PBCInDataStorageRead1/1 -> MATLAB Function/1(u)
  Bus Creator/1 -> Subsystem1/3(PbcIn)
  Demux/32 -> PBCOutFaultStatus_32/1
  Data Type Conversion13/1 -> Bus Creator/14  "WheelPressureReliabilityFrontLeft"
  Demux/12 -> PBCOutFaultStatus_12/1
  Data Type Conversion26/1 -> Bus Creator/27  "WheelPulseRearLeft"
  Data Type Conversion64/1 -> PBCOutOfSpecMsg/1
  Data Type Conversion53/1 -> PBCOutMotorCommandLeft/1
  PBCInHpsAcknowledge/1 -> Data Type Conversion33/1
  PBCInMotorDriverStateLeft/1 -> Data Type Conversion6/1
  Demux/28 -> PBCOutFaultStatus_28/1
  Ground/1 -> FTarR/1
  PBCInRollerBenchActive/1 -> Data Type Conversion32/1
  Data Type Conversion14/1 -> Bus Creator/15  "WheelPressureReliabilityFrontRight"
  Data Type Conversion24/1 -> Bus Creator/25  "WheelPulseFrontLeft"
  Bus Selector/12 -> Data Type Conversion59/1  "<DiagActuationCounterLeft>"

== system APB_Model0_v03_Test/HstEcu/PBC/Subsystem/Subsystem1/Subsystem ==
  PBCInMotorCurrentLeft_1ms : Inport
  Rate Transition11 : RateTransition  OutPortSampleTime=0.01
      settings: AttributesFormatString=%<OutPortSampleTime>
  Scope12 : Scope
  Unit Delay{18..26} (9 alike) : UnitDelay  SampleTime=0.001  HasFrameUpgradeWarning=on
  Vector Concatenate : Concatenate  NumInputs=10
  Out1 : Outport
  wires:
  Vector Concatenate/1 -> Rate Transition11/1
  Unit Delay18/1 -> Vector Concatenate/2, Unit Delay19/1
  Unit Delay20/1 -> Vector Concatenate/4, Unit Delay21/1
  Unit Delay26/1 -> Vector Concatenate/10
  PBCInMotorCurrentLeft_1ms/1 -> Vector Concatenate/1, Scope12/1, Unit Delay18/1
  Unit Delay19/1 -> Vector Concatenate/3, Unit Delay20/1
  Unit Delay22/1 -> Vector Concatenate/6, Unit Delay23/1
  Unit Delay24/1 -> Vector Concatenate/8, Unit Delay25/1
  Unit Delay25/1 -> Vector Concatenate/9, Unit Delay26/1
  Unit Delay23/1 -> Vector Concatenate/7, Unit Delay24/1
  Unit Delay21/1 -> Vector Concatenate/5, Unit Delay22/1
  Rate Transition11/1 -> Out1/1

== system APB_Model0_v03_Test/HstEcu/PBC/Subsystem/Subsystem1/Subsystem4 ==
  note: Invert the order of current signals. From K9 to K0
  PBCInMotorCurrentLeft_1ms : Inport
  Rate Transition : RateTransition  OutPortSampleTime=0.01
  Scope12 : Scope
  Unit Delay{18..26} (9 alike) : UnitDelay  SampleTime=0.001  HasFrameUpgradeWarning=on
  Vector Concatenate : Concatenate  NumInputs=10
  Out1 : Outport
  wires:
  Unit Delay26/1 -> Vector Concatenate/1
  Unit Delay25/1 -> Vector Concatenate/2, Unit Delay26/1
  Unit Delay24/1 -> Vector Concatenate/3, Unit Delay25/1
  Unit Delay23/1 -> Vector Concatenate/4, Unit Delay24/1
  Unit Delay22/1 -> Vector Concatenate/5, Unit Delay23/1
  Unit Delay21/1 -> Vector Concatenate/6, Unit Delay22/1
  Unit Delay20/1 -> Vector Concatenate/7, Unit Delay21/1
  Unit Delay19/1 -> Vector Concatenate/8, Unit Delay20/1
  Unit Delay18/1 -> Vector Concatenate/9, Unit Delay19/1
  PBCInMotorCurrentLeft_1ms/1 -> Vector Concatenate/10, Scope12/1, Unit Delay18/1
  Vector Concatenate/1 -> Rate Transition/1
  Rate Transition/1 -> Out1/1

== system APB_Model0_v03_Test/HstEcu/PBC/Subsystem/Subsystem2/Subsystem ==
  PBCInMotorCurrentLeft_1ms : Inport
  Rate Transition11 : RateTransition  OutPortSampleTime=0.01
      settings: AttributesFormatString=%<OutPortSampleTime>
  Scope12 : Scope
  Unit Delay{18..26} (9 alike) : UnitDelay  SampleTime=0.001  HasFrameUpgradeWarning=on
  Vector Concatenate : Concatenate  NumInputs=10
  Out1 : Outport
  wires:
  Rate Transition11/1 -> Out1/1
  Unit Delay21/1 -> Unit Delay22/1, Vector Concatenate/5
  Unit Delay23/1 -> Unit Delay24/1, Vector Concatenate/7
  Unit Delay25/1 -> Unit Delay26/1, Vector Concatenate/9
  Unit Delay24/1 -> Unit Delay25/1, Vector Concatenate/8
  Unit Delay22/1 -> Unit Delay23/1, Vector Concatenate/6
  Unit Delay19/1 -> Unit Delay20/1, Vector Concatenate/3
  PBCInMotorCurrentLeft_1ms/1 -> Unit Delay18/1, Scope12/1, Vector Concatenate/1
  Unit Delay26/1 -> Vector Concatenate/10
  Unit Delay20/1 -> Unit Delay21/1, Vector Concatenate/4
  Unit Delay18/1 -> Unit Delay19/1, Vector Concatenate/2
  Vector Concatenate/1 -> Rate Transition11/1

== system APB_Model0_v03_Test/HstEcu/PBC/Subsystem/Subsystem2/Subsystem4 ==
  note: Invert the order of current signals. From K9 to K0
  PBCInMotorCurrentLeft_1ms : Inport
  Rate Transition : RateTransition  OutPortSampleTime=0.01
  Scope12 : Scope
  Unit Delay{18..26} (9 alike) : UnitDelay  SampleTime=0.001  HasFrameUpgradeWarning=on
  Vector Concatenate : Concatenate  NumInputs=10
  Out1 : Outport
  wires:
  Rate Transition/1 -> Out1/1
  Vector Concatenate/1 -> Rate Transition/1
  PBCInMotorCurrentLeft_1ms/1 -> Unit Delay18/1, Scope12/1, Vector Concatenate/10
  Unit Delay18/1 -> Unit Delay19/1, Vector Concatenate/9
  Unit Delay19/1 -> Unit Delay20/1, Vector Concatenate/8
  Unit Delay20/1 -> Unit Delay21/1, Vector Concatenate/7
  Unit Delay21/1 -> Unit Delay22/1, Vector Concatenate/6
  Unit Delay22/1 -> Unit Delay23/1, Vector Concatenate/5
  Unit Delay23/1 -> Unit Delay24/1, Vector Concatenate/4
  Unit Delay24/1 -> Unit Delay25/1, Vector Concatenate/3
  Unit Delay25/1 -> Unit Delay26/1, Vector Concatenate/2
  Unit Delay26/1 -> Vector Concatenate/1

== system APB_Model0_v03_Test/HstEcu/PBC/Subsystem/Subsystem3/Subsystem ==
  PBCInMotorCurrentLeft_1ms : Inport
  Rate Transition11 : RateTransition  OutPortSampleTime=0.01
      settings: AttributesFormatString=%<OutPortSampleTime>
  Scope12 : Scope
  Unit Delay{18..26} (9 alike) : UnitDelay  SampleTime=0.001  HasFrameUpgradeWarning=on
  Vector Concatenate : Concatenate  NumInputs=10
  Out1 : Outport
  wires:
  Vector Concatenate/1 -> Rate Transition11/1
  Unit Delay18/1 -> Vector Concatenate/2, Unit Delay19/1
  Unit Delay20/1 -> Vector Concatenate/4, Unit Delay21/1
  Unit Delay26/1 -> Vector Concatenate/10
  PBCInMotorCurrentLeft_1ms/1 -> Vector Concatenate/1, Scope12/1, Unit Delay18/1
  Unit Delay19/1 -> Vector Concatenate/3, Unit Delay20/1
  Unit Delay22/1 -> Vector Concatenate/6, Unit Delay23/1
  Unit Delay24/1 -> Vector Concatenate/8, Unit Delay25/1
  Unit Delay25/1 -> Vector Concatenate/9, Unit Delay26/1
  Unit Delay23/1 -> Vector Concatenate/7, Unit Delay24/1
  Unit Delay21/1 -> Vector Concatenate/5, Unit Delay22/1
  Rate Transition11/1 -> Out1/1

== system APB_Model0_v03_Test/HstEcu/PBC/Subsystem/Subsystem3/Subsystem4 ==
  note: Invert the order of current signals. From K9 to K0
  PBCInMotorCurrentLeft_1ms : Inport
  Rate Transition : RateTransition  OutPortSampleTime=0.01
  Scope12 : Scope
  Unit Delay{18..26} (9 alike) : UnitDelay  SampleTime=0.001  HasFrameUpgradeWarning=on
  Vector Concatenate : Concatenate  NumInputs=10
  Out1 : Outport
  wires:
  Unit Delay26/1 -> Vector Concatenate/1
  Unit Delay25/1 -> Vector Concatenate/2, Unit Delay26/1
  Unit Delay24/1 -> Vector Concatenate/3, Unit Delay25/1
  Unit Delay23/1 -> Vector Concatenate/4, Unit Delay24/1
  Unit Delay22/1 -> Vector Concatenate/5, Unit Delay23/1
  Unit Delay21/1 -> Vector Concatenate/6, Unit Delay22/1
  Unit Delay20/1 -> Vector Concatenate/7, Unit Delay21/1
  Unit Delay19/1 -> Vector Concatenate/8, Unit Delay20/1
  Unit Delay18/1 -> Vector Concatenate/9, Unit Delay19/1
  PBCInMotorCurrentLeft_1ms/1 -> Vector Concatenate/10, Scope12/1, Unit Delay18/1
  Vector Concatenate/1 -> Rate Transition/1
  Rate Transition/1 -> Out1/1

== system APB_Model0_v03_Test/HstEcu/PBC/Subsystem/Subsystem4/Subsystem ==
  PBCInMotorCurrentLeft_1ms : Inport
  Rate Transition11 : RateTransition  OutPortSampleTime=0.01
      settings: AttributesFormatString=%<OutPortSampleTime>
  Scope12 : Scope
  Unit Delay{18..26} (9 alike) : UnitDelay  SampleTime=0.001  HasFrameUpgradeWarning=on
  Vector Concatenate : Concatenate  NumInputs=10
  Out1 : Outport
  wires:
  Rate Transition11/1 -> Out1/1
  Unit Delay21/1 -> Unit Delay22/1, Vector Concatenate/5
  Unit Delay23/1 -> Unit Delay24/1, Vector Concatenate/7
  Unit Delay25/1 -> Unit Delay26/1, Vector Concatenate/9
  Unit Delay24/1 -> Unit Delay25/1, Vector Concatenate/8
  Unit Delay22/1 -> Unit Delay23/1, Vector Concatenate/6
  Unit Delay19/1 -> Unit Delay20/1, Vector Concatenate/3
  PBCInMotorCurrentLeft_1ms/1 -> Unit Delay18/1, Scope12/1, Vector Concatenate/1
  Unit Delay26/1 -> Vector Concatenate/10
  Unit Delay20/1 -> Unit Delay21/1, Vector Concatenate/4
  Unit Delay18/1 -> Unit Delay19/1, Vector Concatenate/2
  Vector Concatenate/1 -> Rate Transition11/1
